simulink model "furuta_lab10"  (R2018a)
settings: Solver=VariableStepAuto  StartTime=0.0  StopTime=20  RelTol=1e-3
libraries: cstblocks x2
settings Model: Creator=ayush2  LastModifiedBy=ayush2

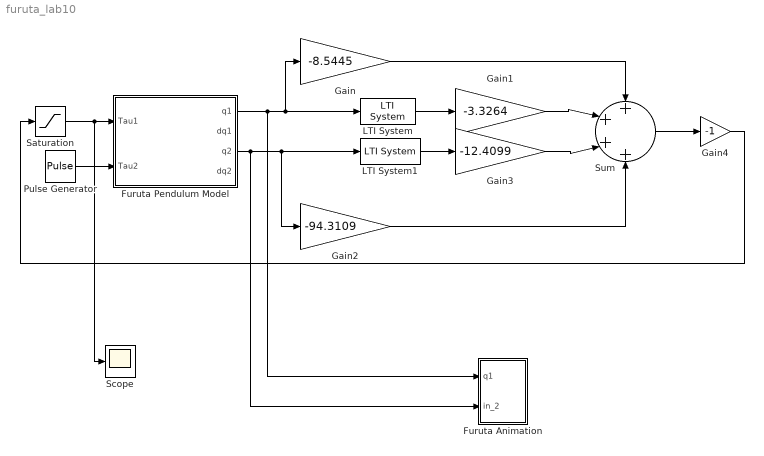
== system furuta_lab10 ==
  Furuta Animation : Subsystem
  Furuta Pendulum Model : Subsystem  mask{par=[0.0363 0.0306 0.0356 0.0260 0.3829], g=9.804, init=[0 0 0 0]}
      mask prompts: par "parameters"; g "acceleration of gravity"; init "Initial Conditions"
  Gain : Gain  Gain=-8.5445
  Gain1 : Gain  Gain=-3.3264
  Gain2 : Gain  Gain=-94.3109
  Gain3 : Gain  Gain=-12.4099
  Gain4 : Gain  Gain=-1
  LTI System : cstblocks/LTI System  sys=difftf  IC=[]
  LTI System1 : cstblocks/LTI System  sys=difftf  IC=[]
  Pulse Generator : DiscretePulseGenerator  PulseType=Time based  Amplitude=3  Period=4  PulseWidth=4  PhaseDelay=4
  Saturation : Saturate  UpperLimit=10  LowerLimit=-10
  Scope : Scope
  Sum : Sum  Inputs=++++
  wires:
  Saturation/1 -> Scope/1, Furuta Pendulum Model/1(Tau1)
  Furuta Pendulum Model/3(q2) -> Furuta Animation/2(in_2), Gain2/1, LTI System1/1
  Furuta Pendulum Model/1(q1) -> Furuta Animation/1(q1), Gain/1, LTI System/1
  LTI System/1 -> Gain1/1
  LTI System1/1 -> Gain3/1
  Gain/1 -> Sum/1
  Gain1/1 -> Sum/2
  Gain3/1 -> Sum/3
  Gain2/1 -> Sum/4
  Sum/1 -> Gain4/1
  Gain4/1 -> Saturation/1
  Pulse Generator/1 -> Furuta Pendulum Model/2(Tau2)

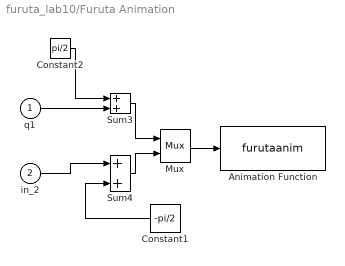
== system furuta_lab10/Furuta Animation ==
  q1 : Inport
  in_2 : Inport  Port=2
  Animation Function : S-Function  FunctionName=furutaanim  Parameters=0.05  SFunctionDeploymentMode=off  EnableBusSupport=off
      settings: DeleteFcn=if ~isempty(findobj('type','figure','name','dblpend1 Animation'));close('dblpend1 Animation'); end;
  Constant1 : Constant  Value=-pi/2
  Constant2 : Constant  Value=pi/2
  Mux : Mux  Inputs=2
  Sum3 : Sum  SaturateOnIntegerOverflow=on  InputSameDT=on  OutDataTypeStr=Inherit: Same as first input
  Sum4 : Sum  SaturateOnIntegerOverflow=on  InputSameDT=on  OutDataTypeStr=Inherit: Same as first input
  wires:
  in_2/1 -> Sum4/1
  Constant1/1 -> Sum4/2
  Mux/1 -> Animation Function/1
  Sum4/1 -> Mux/2
  Sum3/1 -> Mux/1
  Constant2/1 -> Sum3/1
  q1/1 -> Sum3/2

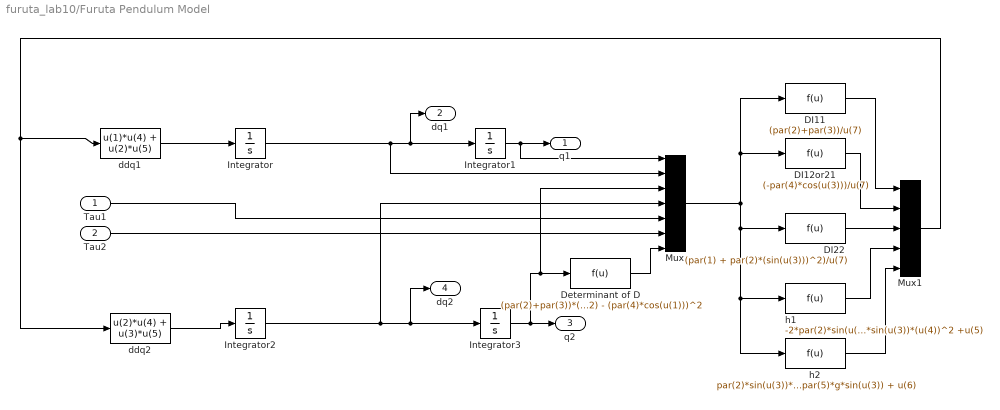
== system furuta_lab10/Furuta Pendulum Model ==
  Tau1 : Inport
  Tau2 : Inport  Port=2
  DI11 : Fcn  Expr=(par(2)+par(3))/u(7)
  DI12or21 : Fcn  Expr=(-par(4)*cos(u(3)))/u(7)
  DI22 : Fcn  Expr=(par(1) + par(2)*(sin(u(3)))^2)/u(7)
  Determinant of D : Fcn  Expr=(par(2)+par(3))*(par(1) + par(2)*(sin(u(1)))^2) - (par(4)*cos(u(1)))^2
  Integrator : Integrator  InitialCondition=init(2)
  Integrator1 : Integrator  InitialCondition=init(1)
  Integrator2 : Integrator  InitialCondition=init(4)
  Integrator3 : Integrator  InitialCondition=init(3)
  Mux : Mux  Inputs=7
  Mux1 : Mux  Inputs=5
  ddq1 : Fcn  Expr=u(1)*u(4) + u(2)*u(5)
  ddq2 : Fcn  Expr=u(2)*u(4) + u(3)*u(5)
  h1 : Fcn  Expr=-2*par(2)*sin(u(3))*cos(u(3))*u(2)*u(4)+par(4)*sin(u(3))*(u(4))^2 +u(5)
  h2 : Fcn  Expr=par(2)*sin(u(3))*cos(u(3))*(u(2))^2 + par(5)*g*sin(u(3)) + u(6)
  q1 : Outport
  dq1 : Outport  Port=2
  q2 : Outport  Port=3
  dq2 : Outport  Port=4
  wires:
  Integrator3/1 -> q2/1, Determinant of D/1, Mux/3
  Integrator1/1 -> q1/1, Mux/1
  Integrator/1 -> Integrator1/1, dq1/1, Mux/2
  Integrator2/1 -> Integrator3/1, dq2/1, Mux/4
  Tau2/1 -> Mux/6
  Tau1/1 -> Mux/5
  Mux/1 -> h2/1, h1/1, DI22/1, DI11/1, DI12or21/1
  DI22/1 -> Mux1/3
  h1/1 -> Mux1/4
  h2/1 -> Mux1/5
  DI12or21/1 -> Mux1/2
  DI11/1 -> Mux1/1
  Mux1/1 -> ddq2/1, ddq1/1
  ddq2/1 -> Integrator2/1
  ddq1/1 -> Integrator/1
  Determinant of D/1 -> Mux/7
